simulink model "mass_SPRING_DAMPER"  (R2017b)
settings: Solver=ode4  StartTime=0.0  StopTime=50  FixedStep=0.1  RelTol=1e-3
values from neighbouring files (symbols this model uses):
  k1 = 1    [lab5.m]
undefined symbols (not defined in the file or in its folder): k2, k3, m1, m2
settings Model: Creator=ArsalanBangash  LastModifiedBy=ArsalanBangash

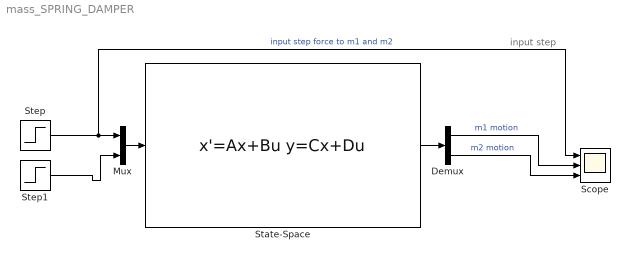
== system mass_SPRING_DAMPER ==
  note: input step
  Demux : Demux  Outputs=2
  Mux : Mux  Inputs=2
  Scope : Scope  NumInputPorts=3
  State-Space : StateSpace  A=[ -(k1+k3)/m2 0 k2/m2 0;0 1 0 0;0 0 0 1; k1/m1 0 -(k1+k2)/m1 0]  B=[0 0; 1/m1 0; 0 0 ;0 1/m2]  C=[1 0 0 0 ; 0 0 1 0]  D=[0 0; 0 0 ]  InitialCondition=0
  Step : Step  Time=2  SampleTime=0
  Step1 : Step  Time=5  SampleTime=0
  wires:
  Mux/1 -> State-Space/1
  State-Space/1 -> Demux/1
  Step/1 -> Scope/1, Mux/1  "input step force to m1 and m2"
  Step1/1 -> Mux/2
  Demux/2 -> Scope/3  "m2 motion"
  Demux/1 -> Scope/2  "m1 motion"
